simulink model "question_10"  (Simulink 5.0)
settings: Solver=ode45  StartTime=0.0  StopTime=1.0  FixedStep=0.001  RelTol=1e-12
values from neighbouring files (symbols this model uses):
  K0 = K(2:end)    [QUESTION.M]
  Ki = K(1)    [QUESTION.M]
  Nx = Nxu(1:n, :)    [QUESTION.M]
  ssobs = ss(ssplant.a-L*ssplant.c, [L ssplant.b-L*ssplant.d], eye(n), 0)    [QUESTION.M]
  ssplant_aug = ss(ssplant.a, ssplant.b, [ssplant.c; zeros(m, n)], [ssplant.d; eye(m)])    [QUESTION.M]
settings Model: LastModifiedBy=Administrator  OptimizeBlockIOStorage=off

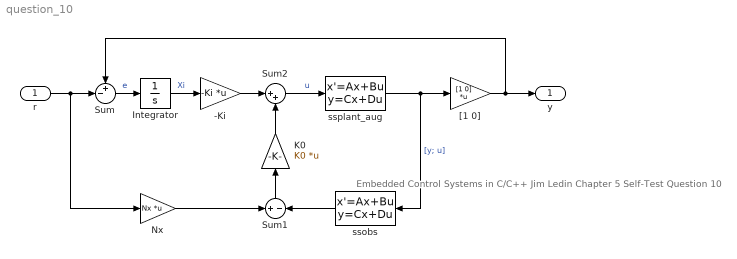
== system question_10 ==
  note: Embedded Control Systems in C/C++
      | Jim Ledin
      | Chapter 5 Self-Test Question 10
  r : Inport
  -Ki : Gain  Gain=-Ki  Multiplication=Matrix(K*u)  SaturateOnIntegerOverflow=on
  Integrator : Integrator  UpperSaturationLimit=0.03  LowerSaturationLimit=-0.03
  K0 : Gain  Orientation=up  Gain=K0  Multiplication=Matrix(K*u)  SaturateOnIntegerOverflow=on
  Nx : Gain  Gain=Nx  Multiplication=Matrix(K*u)  SaturateOnIntegerOverflow=on
  Sum : Sum  Inputs=+-|  SaturateOnIntegerOverflow=on
  Sum1 : Sum  Orientation=up  Inputs=+|-  SaturateOnIntegerOverflow=on
  Sum2 : Sum  Inputs=|++  SaturateOnIntegerOverflow=on
  "[1 0]" : Gain  Gain=[1 0]  Multiplication=Matrix(K*u)  SaturateOnIntegerOverflow=on
  ssobs : StateSpace  Orientation=left  A=ssobs.a  B=ssobs.b  C=ssobs.c  D=ssobs.d
  ssplant_aug : StateSpace  A=ssplant_aug.a  B=ssplant_aug.b  C=ssplant_aug.c  D=ssplant_aug.d
  y : Outport
  wires:
  Nx/1 -> Sum1/1
  Sum1/1 -> K0/1
  Sum/1 -> Integrator/1  "e"
  Integrator/1 -> -Ki/1  "Xi"
  -Ki/1 -> Sum2/1
  K0/1 -> Sum2/2
  Sum2/1 -> ssplant_aug/1  "u"
  ssplant_aug/1 -> ssobs/1, "[1 0]"/1  "[y; u]"
  ssobs/1 -> Sum1/2
  r/1 -> Nx/1, Sum/2
  "[1 0]"/1 -> y/1, Sum/1
